simulink model "FullCarLateral"  (R2023b)
settings: Solver=FixedStepAuto  StartTime=0.0  StopTime=30  FixedStep=dt  MaxStep=0.001  RelTol=1e-3
model workspace (MAT data in the model file):
  AMU : Simulink.Signal (value not decoded)
  EPSILON : Simulink.Signal (value not decoded)
  FZO : Simulink.Signal (value not decoded)
  LCX : Simulink.Signal (value not decoded)
  LCY : Simulink.Signal (value not decoded)
  LCZ : Simulink.Signal (value not decoded)
  LEX : Simulink.Signal (value not decoded)
  LEY : Simulink.Signal (value not decoded)
  LFZO : Simulink.Signal (value not decoded)
  LHX : Simulink.Signal (value not decoded)
  LHY : Simulink.Signal (value not decoded)
  LKXKAPPA : Simulink.Signal (value not decoded)
  LKYALPHA : Simulink.Signal (value not decoded)
  LKYGAMMA : Simulink.Signal (value not decoded)
  LKZGAMMA : Simulink.Signal (value not decoded)
  LMR : Simulink.Signal (value not decoded)
  LMUV : Simulink.Signal (value not decoded)
  LMUX : Simulink.Signal (value not decoded)
  LMUXAST : Simulink.Signal (value not decoded)
  LMUXPRIME : Simulink.Signal (value not decoded)
  LMUY : Simulink.Signal (value not decoded)
  LMUYAST : Simulink.Signal (value not decoded)
  LMUYPRIME : Simulink.Signal (value not decoded)
  LMX : Simulink.Signal (value not decoded)
  LMY : Simulink.Signal (value not decoded)
  LS : Simulink.Signal (value not decoded)
  LT : Simulink.Signal (value not decoded)
  LVX : Simulink.Signal (value not decoded)
  LVY : Simulink.Signal (value not decoded)
  LVYKAPPA : Simulink.Signal (value not decoded)
  LXALPHA : Simulink.Signal (value not decoded)
  LYKAPPA : Simulink.Signal (value not decoded)
  PCX1 : Simulink.Signal (value not decoded)
  PCY1 : Simulink.Signal (value not decoded)
  PDX1 : Simulink.Signal (value not decoded)
  PDX2 : Simulink.Signal (value not decoded)
  PDX3 : Simulink.Signal (value not decoded)
  PDY1 : Simulink.Signal (value not decoded)
  PDY2 : Simulink.Signal (value not decoded)
  PDY3 : Simulink.Signal (value not decoded)
  PEX1 : Simulink.Signal (value not decoded)
  PEX2 : Simulink.Signal (value not decoded)
  PEX3 : Simulink.Signal (value not decoded)
  PEX4 : Simulink.Signal (value not decoded)
  PEY1 : Simulink.Signal (value not decoded)
  PEY2 : Simulink.Signal (value not decoded)
  PEY3 : Simulink.Signal (value not decoded)
  PEY4 : Simulink.Signal (value not decoded)
  PEY5 : Simulink.Signal (value not decoded)
  PHX1 : Simulink.Signal (value not decoded)
  PHX2 : Simulink.Signal (value not decoded)
  PHY1 : Simulink.Signal (value not decoded)
  PHY2 : Simulink.Signal (value not decoded)
  PKX1 : Simulink.Signal (value not decoded)
  PKX2 : Simulink.Signal (value not decoded)
  PKX3 : Simulink.Signal (value not decoded)
  PKY1 : Simulink.Signal (value not decoded)
  PKY2 : Simulink.Signal (value not decoded)
  PKY3 : Simulink.Signal (value not decoded)
  PKY4 : Simulink.Signal (value not decoded)
  PKY5 : Simulink.Signal (value not decoded)
  PKY6 : Simulink.Signal (value not decoded)
  PKY7 : Simulink.Signal (value not decoded)
  PVX1 : Simulink.Signal (value not decoded)
  PVX2 : Simulink.Signal (value not decoded)
  PVY1 : Simulink.Signal (value not decoded)
  PVY2 : Simulink.Signal (value not decoded)
  PVY3 : Simulink.Signal (value not decoded)
  PVY4 : Simulink.Signal (value not decoded)
  QBZ1 : Simulink.Signal (value not decoded)
  QBZ10 : Simulink.Signal (value not decoded)
  QBZ2 : Simulink.Signal (value not decoded)
  QBZ3 : Simulink.Signal (value not decoded)
  QBZ5 : Simulink.Signal (value not decoded)
  QBZ6 : Simulink.Signal (value not decoded)
  QBZ9 : Simulink.Signal (value not decoded)
  QCZ1 : Simulink.Signal (value not decoded)
  QDZ1 : Simulink.Signal (value not decoded)
  QDZ10 : Simulink.Signal (value not decoded)
  QDZ11 : Simulink.Signal (value not decoded)
  QDZ2 : Simulink.Signal (value not decoded)
  QDZ3 : Simulink.Signal (value not decoded)
  QDZ4 : Simulink.Signal (value not decoded)
  QDZ6 : Simulink.Signal (value not decoded)
  QDZ7 : Simulink.Signal (value not decoded)
  QDZ8 : Simulink.Signal (value not decoded)
  QDZ9 : Simulink.Signal (value not decoded)
  QEZ1 : Simulink.Signal (value not decoded)
  QEZ2 : Simulink.Signal (value not decoded)
  QEZ3 : Simulink.Signal (value not decoded)
  QEZ4 : Simulink.Signal (value not decoded)
  QEZ5 : Simulink.Signal (value not decoded)
  QHZ1 : Simulink.Signal (value not decoded)
  QHZ2 : Simulink.Signal (value not decoded)
  QHZ3 : Simulink.Signal (value not decoded)
  QHZ4 : Simulink.Signal (value not decoded)
  QSX1 : Simulink.Signal (value not decoded)
  QSX2 : Simulink.Signal (value not decoded)
  QSX3 : Simulink.Signal (value not decoded)
  QX1 : Simulink.Signal (value not decoded)
  QX2 : Simulink.Signal (value not decoded)
  QX3 : Simulink.Signal (value not decoded)
  QX4 : Simulink.Signal (value not decoded)
  QX5 : Simulink.Signal (value not decoded)
  QX6 : Simulink.Signal (value not decoded)
  RBX1 : Simulink.Signal (value not decoded)
  RBX2 : Simulink.Signal (value not decoded)
  RBX3 : Simulink.Signal (value not decoded)
  RBY1 : Simulink.Signal (value not decoded)
  RBY2 : Simulink.Signal (value not decoded)
  RBY3 : Simulink.Signal (value not decoded)
  RBY4 : Simulink.Signal (value not decoded)
  RCX1 : Simulink.Signal (value not decoded)
  RCY1 : Simulink.Signal (value not decoded)
  REX1 : Simulink.Signal (value not decoded)
  REX2 : Simulink.Signal (value not decoded)
  REY1 : Simulink.Signal (value not decoded)
  REY2 : Simulink.Signal (value not decoded)
  RHX1 : Simulink.Signal (value not decoded)
  RHY1 : Simulink.Signal (value not decoded)
  RHY2 : Simulink.Signal (value not decoded)
  RO : Simulink.Signal (value not decoded)
  RVY1 : Simulink.Signal (value not decoded)
  RVY2 : Simulink.Signal (value not decoded)
  RVY3 : Simulink.Signal (value not decoded)
  RVY4 : Simulink.Signal (value not decoded)
  RVY5 : Simulink.Signal (value not decoded)
  RVY6 : Simulink.Signal (value not decoded)
  SSZ1 : Simulink.Signal (value not decoded)
  SSZ2 : Simulink.Signal (value not decoded)
  SSZ3 : Simulink.Signal (value not decoded)
  SSZ4 : Simulink.Signal (value not decoded)
  VCX : Simulink.Signal (value not decoded)
  ZETA0 : Simulink.Signal (value not decoded)
  ZETA1 : Simulink.Signal (value not decoded)
  ZETA2 : Simulink.Signal (value not decoded)
  ZETA3 : Simulink.Signal (value not decoded)
  ZETA4 : Simulink.Signal (value not decoded)
  ZETA5 : Simulink.Signal (value not decoded)
  ZETA6 : Simulink.Signal (value not decoded)
  ZETA7 : Simulink.Signal (value not decoded)
  ZETA8 : Simulink.Signal (value not decoded)
values from neighbouring files (symbols this model uses):
  A = load('PSS LATERAL FORCE COEFFS.mat').A    [FullCarLateralParams.m]
  B = load('PSS ALIGNING TORQUE COEFFS.mat').B    [FullCarLateralParams.m]
  b = 0.085    [FullCarLateralParams.m]
  C = load('COMBINED OVERTURNING MOMENT COEFFS.mat').C    [FullCarLateralParams.m]
  c_roll = 0.1    [FullCarLateralParams.m]
  cD = 1.23    [FullCarLateralParams.m]
  cL = 3.71    [FullCarLateralParams.m]
  D = load('PLS LONGITUDINAL FORCE COEFFS.mat').D    [FullCarLateralParams.m]
  dt = 0.001    [FullCarLateralParams.m]
  E = load('COMBINED LONGITUDINAL FORCE COEFFS.mat').E    [FullCarLateralParams.m]
  e_FL = atan(tf/lf)    [FullCarLateralParams.m]
  e_FR = atan(lf/tf)    [FullCarLateralParams.m]
  e_RL = atan(lr/tr)    [FullCarLateralParams.m]
  e_RR = atan(tr/lr)    [FullCarLateralParams.m]
  F = load('COMBINED LATERAL FORCE COEFFS.mat').F    [FullCarLateralParams.m]
  frontalA = 1    [FullCarLateralParams.m]
  g = 9.81    [FullCarLateralParams.m]
  G = load('COMBINED ALIGNING TORQUE COEFFS.mat').G    [FullCarLateralParams.m]
  gearboxEff = 0.95    [FullCarLateralParams.m]
  GR = 11.86    [FullCarLateralParams.m]
  hCG = 0.2    [FullCarLateralParams.m]
  Ix_wheel = (0.07829 + Ix_motor*GR*GR) * Ix_wheel_factor    (= 0.1168307304)    [FullCarLateralParams.m]
  Iz_vehicle = 125    [FullCarLateralParams.m]
  lf = wb - lr    (= 0.755)    [FullCarLateralParams.m]
  lowpassT = 0.05    [FullCarLateralParams.m]
  lr = 0.78    [FullCarLateralParams.m]
  m = 250    [FullCarLateralParams.m]
  motorOmegaLimit = 2094    [FullCarLateralParams.m]
  R_FL = sqrt(tf^2 + lf^2)    [FullCarLateralParams.m]
  R_FR = R_FL    [FullCarLateralParams.m]
  R_RL = sqrt(tr^2 + lr^2)    [FullCarLateralParams.m]
  R_RR = R_RL    [FullCarLateralParams.m]
  R_wheel = 0.2    [FullCarLateralParams.m]
  rho = 1.293    [FullCarLateralParams.m]
  tireFactor_X_Accel = 0.6    [FullCarLateralParams.m]
  tireFactor_X_Brake = 0.6    [FullCarLateralParams.m]
  tireFactor_Y = 1    [FullCarLateralParams.m]
  TLLTD = 0.5    [FullCarLateralParams.m]
  tr = trackWidth / 2    (= 0.6)    [FullCarLateralParams.m]
  trackWidth = 1.2    [FullCarLateralParams.m]
  wb = 1.535    [FullCarLateralParams.m]
  wheelSideBrakeFactor = 1    [FullCarLateralParams.m]
undefined symbols (not defined in the file or in its folder): trackReference
libraries: simulink_extras x11, eeGeneralControl x3, slpidlib x2, simulink x2
(part 3 of 6)

== system FullCarLateral/Car/Tire Model Pacejka 5.2/Subsystem1 ==
  FX : Inport
  If : If  IfExpression=u1 >= 0
  If Action Subsystem : Subsystem  TreatAsAtomicUnit=on
  If Action Subsystem1 : Subsystem  TreatAsAtomicUnit=on
  Merge : Merge
  FX_W FR : Outport
  wires:
  If Action Subsystem1/1(Out1) -> Merge/2
  If Action Subsystem/1(Out1) -> Merge/1
  If/2 -> If Action Subsystem1/Action
  Merge/1 -> FX_W FR/1  "FX_W FL"
  FX/1 -> If Action Subsystem/1(FX), If Action Subsystem1/1(FX), If/1
  If/1 -> If Action Subsystem/Action

== system FullCarLateral/Car/Tire Model Pacejka 5.2/Subsystem2 ==
  FX : Inport
  If : If  IfExpression=u1 >= 0
  If Action Subsystem : Subsystem  TreatAsAtomicUnit=on
  If Action Subsystem1 : Subsystem  TreatAsAtomicUnit=on
  Merge : Merge
  FX_W RL : Outport
  wires:
  If/1 -> If Action Subsystem/Action
  FX/1 -> If/1, If Action Subsystem1/1(FX), If Action Subsystem/1(FX)
  Merge/1 -> FX_W RL/1  "FX_W FL"
  If/2 -> If Action Subsystem1/Action
  If Action Subsystem/1(Out1) -> Merge/1
  If Action Subsystem1/1(Out1) -> Merge/2

== system FullCarLateral/Car/Tire Model Pacejka 5.2/Subsystem3 ==
  FX : Inport
  If : If  IfExpression=u1 >= 0
  If Action Subsystem : Subsystem  TreatAsAtomicUnit=on
  If Action Subsystem1 : Subsystem  TreatAsAtomicUnit=on
  Merge : Merge
  FX_W RR : Outport
  wires:
  If Action Subsystem1/1(Out1) -> Merge/2
  If Action Subsystem/1(Out1) -> Merge/1
  If/2 -> If Action Subsystem1/Action
  Merge/1 -> FX_W RR/1  "FX_W FL"
  FX/1 -> If Action Subsystem/1(FX), If Action Subsystem1/1(FX), If/1
  If/1 -> If Action Subsystem/Action

== system FullCarLateral/Car/Wheel Dynamics/Subsystem ==
  FX : Inport
  FY : Inport  Port=2
  Add : Sum
  Product : Product
  Product1 : Product
  Product2 : Product
  Sign : Signum
  Sqrt : Sqrt
  F NET : Outport
  wires:
  FX/1 -> Sign/1, Product/2, Product/1
  FY/1 -> Product1/1, Product1/2
  Product/1 -> Add/1
  Product1/1 -> Add/2
  Add/1 -> Sqrt/1
  Sqrt/1 -> Product2/2
  Sign/1 -> Product2/1
  Product2/1 -> F NET/1

== system FullCarLateral/Car/Wheel Dynamics/Subsystem1 ==
  FX : Inport
  FY : Inport  Port=2
  Add : Sum
  Product : Product
  Product1 : Product
  Product2 : Product
  Sign : Signum
  Sqrt : Sqrt
  F NET : Outport
  wires:
  Product2/1 -> F NET/1
  Sign/1 -> Product2/1
  Sqrt/1 -> Product2/2
  Add/1 -> Sqrt/1
  Product1/1 -> Add/2
  Product/1 -> Add/1
  FY/1 -> Product1/2, Product1/1
  FX/1 -> Product/1, Product/2, Sign/1

== system FullCarLateral/Car/Wheel Dynamics/Subsystem2 ==
  FX : Inport
  FY : Inport  Port=2
  Add : Sum
  Product : Product
  Product1 : Product
  Product2 : Product
  Sign : Signum
  Sqrt : Sqrt
  F NET : Outport
  wires:
  FX/1 -> Sign/1, Product/2, Product/1
  FY/1 -> Product1/1, Product1/2
  Product/1 -> Add/1
  Product1/1 -> Add/2
  Add/1 -> Sqrt/1
  Sqrt/1 -> Product2/2
  Sign/1 -> Product2/1
  Product2/1 -> F NET/1

== system FullCarLateral/Car/Wheel Dynamics/Subsystem3 ==
  FX : Inport
  FY : Inport  Port=2
  Add : Sum
  Product : Product
  Product1 : Product
  Product2 : Product
  Sign : Signum
  Sqrt : Sqrt
  F NET : Outport
  wires:
  Product2/1 -> F NET/1
  Sign/1 -> Product2/1
  Sqrt/1 -> Product2/2
  Add/1 -> Sqrt/1
  Product1/1 -> Add/2
  Product/1 -> Add/1
  FY/1 -> Product1/2, Product1/1
  FX/1 -> Product/1, Product/2, Sign/1

== system FullCarLateral/Car/Wheel Dynamics/Subsystem4 ==
  Requested Motor Torque : Inport
  FX Resistance : Inport  Port=2
  Long Corner Vel : Inport  Port=3
  Accel. or Rolling No Slip : Subsystem  TreatAsAtomicUnit=on
  Braking : Subsystem  TreatAsAtomicUnit=on
  Constant : Constant  Value=0
  If : If  IfExpression=u1 >= 0
  Merge : Merge
  Merge1 : Merge
  Switch : Switch  Criteria=u2 > Threshold  SaturateOnIntegerOverflow=off  InputSameDT=off
  Wheel Omega : Outport
  Constrained Motor Torque : Outport  Port=2
  wires:
  Requested Motor Torque/1 -> Braking/1(Requested Motor Torque), Accel. or Rolling No Slip/1(Requested Motor Torque), If/1
  If/1 -> Accel. or Rolling No Slip/Action
  If/2 -> Braking/Action
  FX Resistance/1 -> Braking/2(FX Resistance), Accel. or Rolling No Slip/2(FX Resistance)
  Long Corner Vel/1 -> Accel. or Rolling No Slip/3(Long Corner Vel)
  Accel. or Rolling No Slip/1(Wheel Omega) -> Merge/1
  Braking/1(Wheel Omega) -> Merge/2
  Accel. or Rolling No Slip/2(Constrained Motor Torque) -> Merge1/1
  Braking/2(Constrained Motor Torque) -> Merge1/2
  Merge1/1 -> Constrained Motor Torque/1
  Merge/1 -> Switch/2, Switch/1
  Switch/1 -> Wheel Omega/1
  Constant/1 -> Switch/3

== system FullCarLateral/Car/Wheel Dynamics/Subsystem5 ==
  Requested Motor Torque : Inport
  FX Resistance : Inport  Port=2
  Long Corner Vel : Inport  Port=3
  Accel. or Rolling No Slip : Subsystem  TreatAsAtomicUnit=on
  Braking : Subsystem  TreatAsAtomicUnit=on
  Constant : Constant  Value=0
  If : If  IfExpression=u1 >= 0
  Merge : Merge
  Merge1 : Merge
  Switch : Switch  Criteria=u2 > Threshold  SaturateOnIntegerOverflow=off  InputSameDT=off
  Wheel Omega : Outport
  Constrained Motor Torque : Outport  Port=2
  wires:
  Merge1/1 -> Constrained Motor Torque/1
  Braking/2(Constrained Motor Torque) -> Merge1/2
  Accel. or Rolling No Slip/2(Constrained Motor Torque) -> Merge1/1
  Braking/1(Wheel Omega) -> Merge/2
  Accel. or Rolling No Slip/1(Wheel Omega) -> Merge/1
  Long Corner Vel/1 -> Accel. or Rolling No Slip/3(Long Corner Vel)
  FX Resistance/1 -> Accel. or Rolling No Slip/2(FX Resistance), Braking/2(FX Resistance)
  If/2 -> Braking/Action
  If/1 -> Accel. or Rolling No Slip/Action
  Requested Motor Torque/1 -> If/1, Accel. or Rolling No Slip/1(Requested Motor Torque), Braking/1(Requested Motor Torque)
  Constant/1 -> Switch/3
  Merge/1 -> Switch/2, Switch/1
  Switch/1 -> Wheel Omega/1

== system FullCarLateral/Car/Wheel Dynamics/Subsystem6 ==
  Requested Motor Torque : Inport
  FX Resistance : Inport  Port=2
  Long Corner Vel : Inport  Port=3
  Accel. or Rolling No Slip : Subsystem  TreatAsAtomicUnit=on
  Braking : Subsystem  TreatAsAtomicUnit=on
  Constant : Constant  Value=0
  If : If  IfExpression=u1 >= 0
  Merge : Merge
  Merge1 : Merge
  Switch : Switch  Criteria=u2 > Threshold  SaturateOnIntegerOverflow=off  InputSameDT=off
  Wheel Omega : Outport
  Constrained Motor Torque : Outport  Port=2
  wires:
  Requested Motor Torque/1 -> Braking/1(Requested Motor Torque), Accel. or Rolling No Slip/1(Requested Motor Torque), If/1
  If/1 -> Accel. or Rolling No Slip/Action
  If/2 -> Braking/Action
  FX Resistance/1 -> Braking/2(FX Resistance), Accel. or Rolling No Slip/2(FX Resistance)
  Long Corner Vel/1 -> Accel. or Rolling No Slip/3(Long Corner Vel)
  Accel. or Rolling No Slip/1(Wheel Omega) -> Merge/1
  Braking/1(Wheel Omega) -> Merge/2
  Accel. or Rolling No Slip/2(Constrained Motor Torque) -> Merge1/1
  Braking/2(Constrained Motor Torque) -> Merge1/2
  Merge1/1 -> Constrained Motor Torque/1
  Constant/1 -> Switch/3
  Merge/1 -> Switch/2, Switch/1
  Switch/1 -> Wheel Omega/1

== system FullCarLateral/Car/Wheel Dynamics/Subsystem7 ==
  Requested Motor Torque : Inport
  FX Resistance : Inport  Port=2
  Long Corner Vel : Inport  Port=3
  Accel. or Rolling No Slip : Subsystem  TreatAsAtomicUnit=on
  Braking : Subsystem  TreatAsAtomicUnit=on
  Constant : Constant  Value=0
  If : If  IfExpression=u1 >= 0
  Merge : Merge
  Merge1 : Merge
  Switch : Switch  Criteria=u2 > Threshold  SaturateOnIntegerOverflow=off  InputSameDT=off
  Wheel Omega : Outport
  Constrained Motor Torque : Outport  Port=2
  wires:
  Merge1/1 -> Constrained Motor Torque/1
  Braking/2(Constrained Motor Torque) -> Merge1/2
  Accel. or Rolling No Slip/2(Constrained Motor Torque) -> Merge1/1
  Braking/1(Wheel Omega) -> Merge/2
  Accel. or Rolling No Slip/1(Wheel Omega) -> Merge/1
  Long Corner Vel/1 -> Accel. or Rolling No Slip/3(Long Corner Vel)
  FX Resistance/1 -> Accel. or Rolling No Slip/2(FX Resistance), Braking/2(FX Resistance)
  If/2 -> Braking/Action
  If/1 -> Accel. or Rolling No Slip/Action
  Requested Motor Torque/1 -> If/1, Accel. or Rolling No Slip/1(Requested Motor Torque), Braking/1(Requested Motor Torque)
  Constant/1 -> Switch/3
  Merge/1 -> Switch/2, Switch/1
  Switch/1 -> Wheel Omega/1

== system FullCarLateral/Car/Wheel Dynamics/Wheel Omega Calc FL1 ==
  Requested Motor Torque : Inport
  FX Resistance : Inport  Port=2
  Add3 : Sum
  Apply Motor Omega Limit Constraint : Subsystem  TreatAsAtomicUnit=on
  Constant12 : Constant  Value=b
  Constant16 : Constant  Value=GR
  Constant20 : Constant  Value=R_wheel
  Data Store Read2 : DataStoreRead  DataStoreName=wheelOmegaFL  IndexOptions=Index vector (dialog)  Indices=1  OutputSizes=1
  Divide : Product  Inputs=*/
  Fcn3 : Fcn  Expr=u/Ix_wheel
  Gain : Gain  Gain=wheelSideBrakeFactor
  Gain14 : Gain  Gain=gearboxEff
  Gain15 : Gain  Gain=dt
  Gain16 : Gain  Gain=GR
  If3 : If  IfExpression=u1 > motorOmegaLimit
  Memory2 : Memory
  No Omega Limit Constraint : Subsystem  TreatAsAtomicUnit=on
  Product15 : Product
  Product16 : Product
  Product20 : Product
  Subtract5 : Sum  Inputs=+--
  Switch : Switch  Criteria=u2 > Threshold  SaturateOnIntegerOverflow=off  InputSameDT=off
  Terminator : Terminator
  wires:
  Product16/1 -> Gain14/1
  Product20/1 -> Subtract5/2
  Requested Motor Torque/1 -> No Omega Limit Constraint/2(Unconstrained Requested Motor Torque), Apply Motor Omega Limit Constraint/1(Requested Motor Torque), Product16/1
  Add3/1 -> Gain16/1, No Omega Limit Constraint/1(Wheel Omega), Product15/2  "Wheel Omega"
  Data Store Read2/1 -> Add3/2  "Previous Wheel Omega"
  Memory2/1 -> Gain15/1
  Subtract5/1 -> Fcn3/1
  Constant20/1 -> Divide/2, Product20/2
  Gain15/1 -> Add3/1  "Delta Wheel Omega"
  Fcn3/1 -> Memory2/1  "Wheel Omega Dot"
  If3/2 -> No Omega Limit Constraint/Action
  Product15/1 -> Subtract5/3
  Constant12/1 -> Product15/1
  Gain14/1 -> Divide/1, Subtract5/1  "Requested Wheel Output Torque"
  Constant16/1 -> Product16/2
  If3/1 -> Apply Motor Omega Limit Constraint/Action
  Gain16/1 -> If3/1  "Motor Omega"
  Switch/1 -> Product20/1, Apply Motor Omega Limit Constraint/2(F_Roll)
  FX Resistance/1 -> Switch/1, Switch/2, Gain/1
  Gain/1 -> Switch/3
  Divide/1 -> Terminator/1  "Linear Force From Motor Torque FL"

== system FullCarLateral/Car/Wheel Dynamics/Wheel Omega Calc FR1 ==
  Requested Motor Torque : Inport
  FX Resistance : Inport  Port=2
  Add3 : Sum
  Apply Motor Omega Limit Constraint : Subsystem  TreatAsAtomicUnit=on
  Constant12 : Constant  Value=b
  Constant16 : Constant  Value=GR
  Constant20 : Constant  Value=R_wheel
  Data Store Read2 : DataStoreRead  DataStoreName=wheelOmegaFR  IndexOptions=Index vector (dialog)  Indices=1  OutputSizes=1
  Fcn3 : Fcn  Expr=u/Ix_wheel
  Gain1 : Gain  Gain=wheelSideBrakeFactor
  Gain14 : Gain  Gain=gearboxEff
  Gain15 : Gain  Gain=dt
  Gain16 : Gain  Gain=GR
  If3 : If  IfExpression=u1 > motorOmegaLimit
  Memory2 : Memory
  No Omega Limit Constraint : Subsystem  TreatAsAtomicUnit=on
  Product15 : Product
  Product16 : Product
  Product20 : Product
  Subtract5 : Sum  Inputs=+--
  Switch1 : Switch  Criteria=u2 > Threshold  SaturateOnIntegerOverflow=off  InputSameDT=off
  wires:
  Gain16/1 -> If3/1  "Motor Omega"
  If3/1 -> Apply Motor Omega Limit Constraint/Action
  Constant16/1 -> Product16/2
  Gain14/1 -> Subtract5/1  "Requested Wheel Output Torque"
  Constant12/1 -> Product15/1
  Product15/1 -> Subtract5/3
  If3/2 -> No Omega Limit Constraint/Action
  Fcn3/1 -> Memory2/1  "Wheel Omega Dot"
  Gain15/1 -> Add3/1  "Delta Wheel Omega"
  Constant20/1 -> Product20/2
  Subtract5/1 -> Fcn3/1
  Memory2/1 -> Gain15/1
  Data Store Read2/1 -> Add3/2  "Previous Wheel Omega"
  Add3/1 -> Product15/2, No Omega Limit Constraint/1(Wheel Omega), Gain16/1  "Wheel Omega"
  Requested Motor Torque/1 -> Product16/1, Apply Motor Omega Limit Constraint/1(Requested Motor Torque), No Omega Limit Constraint/2(Unconstrained Requested Motor Torque)
  Product20/1 -> Subtract5/2
  Product16/1 -> Gain14/1
  Gain1/1 -> Switch1/3
  FX Resistance/1 -> Gain1/1, Switch1/2, Switch1/1
  Switch1/1 -> Product20/1, Apply Motor Omega Limit Constraint/2(F_Roll)

== system FullCarLateral/Car/Wheel Dynamics/Wheel Omega Calc RL1 ==
  Requested Motor Torque : Inport
  FX Resistance : Inport  Port=2
  Add3 : Sum
  Apply Motor Omega Limit Constraint : Subsystem  TreatAsAtomicUnit=on
  Constant12 : Constant  Value=b
  Constant16 : Constant  Value=GR
  Constant20 : Constant  Value=R_wheel
  Data Store Read2 : DataStoreRead  DataStoreName=wheelOmegaRL  IndexOptions=Index vector (dialog)  Indices=1  OutputSizes=1
  Fcn3 : Fcn  Expr=u/Ix_wheel
  Gain : Gain  Gain=wheelSideBrakeFactor
  Gain14 : Gain  Gain=gearboxEff
  Gain15 : Gain  Gain=dt
  Gain16 : Gain  Gain=GR
  If3 : If  IfExpression=u1 > motorOmegaLimit
  Memory2 : Memory
  No Omega Limit Constraint : Subsystem  TreatAsAtomicUnit=on
  Product15 : Product
  Product16 : Product
  Product20 : Product
  Subtract5 : Sum  Inputs=+--
  Switch : Switch  Criteria=u2 > Threshold  SaturateOnIntegerOverflow=off  InputSameDT=off
  wires:
  Product16/1 -> Gain14/1
  Product20/1 -> Subtract5/2
  Requested Motor Torque/1 -> No Omega Limit Constraint/2(Unconstrained Requested Motor Torque), Apply Motor Omega Limit Constraint/1(Requested Motor Torque), Product16/1
  Add3/1 -> Gain16/1, No Omega Limit Constraint/1(Wheel Omega), Product15/2  "Wheel Omega"
  Data Store Read2/1 -> Add3/2  "Previous Wheel Omega"
  Memory2/1 -> Gain15/1
  Subtract5/1 -> Fcn3/1
  Constant20/1 -> Product20/2
  Gain15/1 -> Add3/1  "Delta Wheel Omega"
  Fcn3/1 -> Memory2/1  "Wheel Omega Dot"
  If3/2 -> No Omega Limit Constraint/Action
  Product15/1 -> Subtract5/3
  Constant12/1 -> Product15/1
  Gain14/1 -> Subtract5/1  "Requested Wheel Output Torque"
  Constant16/1 -> Product16/2
  If3/1 -> Apply Motor Omega Limit Constraint/Action
  Gain16/1 -> If3/1  "Motor Omega"
  Gain/1 -> Switch/3
  FX Resistance/1 -> Switch/1, Gain/1, Switch/2
  Switch/1 -> Apply Motor Omega Limit Constraint/2(F_Roll), Product20/1

== system FullCarLateral/Car/Wheel Dynamics/Wheel Omega Calc RR1 ==
  Requested Motor Torque : Inport
  FX Resistance : Inport  Port=2
  Add3 : Sum
  Apply Motor Omega Limit Constraint : Subsystem  TreatAsAtomicUnit=on
  Constant12 : Constant  Value=b
  Constant16 : Constant  Value=GR
  Constant20 : Constant  Value=R_wheel
  Data Store Read2 : DataStoreRead  DataStoreName=wheelOmegaRR  IndexOptions=Index vector (dialog)  Indices=1  OutputSizes=1
  Fcn3 : Fcn  Expr=u/Ix_wheel
  Gain : Gain  Gain=wheelSideBrakeFactor
  Gain14 : Gain  Gain=gearboxEff
  Gain15 : Gain  Gain=dt
  Gain16 : Gain  Gain=GR
  If3 : If  IfExpression=u1 > motorOmegaLimit
  Memory2 : Memory
  No Omega Limit Constraint : Subsystem  TreatAsAtomicUnit=on
  Product15 : Product
  Product16 : Product
  Product20 : Product
  Subtract5 : Sum  Inputs=+--
  Switch : Switch  Criteria=u2 > Threshold  SaturateOnIntegerOverflow=off  InputSameDT=off
  wires:
  Gain16/1 -> If3/1  "Motor Omega"
  If3/1 -> Apply Motor Omega Limit Constraint/Action
  Constant16/1 -> Product16/2
  Gain14/1 -> Subtract5/1  "Requested Wheel Output Torque"
  Constant12/1 -> Product15/1
  Product15/1 -> Subtract5/3
  If3/2 -> No Omega Limit Constraint/Action
  Fcn3/1 -> Memory2/1  "Wheel Omega Dot"
  Gain15/1 -> Add3/1  "Delta Wheel Omega"
  Constant20/1 -> Product20/2
  Subtract5/1 -> Fcn3/1
  Memory2/1 -> Gain15/1
  Data Store Read2/1 -> Add3/2  "Previous Wheel Omega"
  Add3/1 -> Product15/2, No Omega Limit Constraint/1(Wheel Omega), Gain16/1  "Wheel Omega"
  Requested Motor Torque/1 -> Product16/1, Apply Motor Omega Limit Constraint/1(Requested Motor Torque), No Omega Limit Constraint/2(Unconstrained Requested Motor Torque)
  Product20/1 -> Subtract5/2
  Product16/1 -> Gain14/1
  Gain/1 -> Switch/3
  FX Resistance/1 -> Switch/1, Gain/1, Switch/2
  Switch/1 -> Product20/1, Apply Motor Omega Limit Constraint/2(F_Roll)

== system FullCarLateral/Car/Longitudinal Slip/Longitudinal Slip Calc FL/Accel. Calc ==
  Corner Speed : Inport
  Wheel Omega1 : Inport  Port=2
  Action Port : ActionPort  ActionPortLabel=if(u1 > 0)
  Add : Sum  Commented=on
  Constant : Constant  Value=R_wheel
  Constant1 : Constant  Value=inf
  Constant2 : Constant
  Constant3 : Constant  Value=0
  Constant4 : Constant  Commented=on
  Divide : Product  Inputs=*/
  From : From  Commented=on  GotoTag=SL
  From1 : From  Commented=on  GotoTag=SS
  Product : Product
  Product3 : Product  Commented=on
  Product4 : Product  Commented=on
  Sqrt : Sqrt  Commented=on
  Subtract : Sum  Inputs=+-
  Switch : Switch  Criteria=u2 ~= 0  SaturateOnIntegerOverflow=off  InputSameDT=off
  Switch1 : Switch  Criteria=u2 > Threshold  Threshold=1  SaturateOnIntegerOverflow=off  InputSameDT=off
  Switch2 : Switch  Commented=on  Criteria=u2 > Threshold  Threshold=1  SaturateOnIntegerOverflow=off  InputSameDT=off
  Switch3 : Switch  Criteria=u2 > Threshold  SaturateOnIntegerOverflow=off  InputSameDT=off
  SL : Outport
  wires:
  Switch/1 -> Divide/2
  Constant1/1 -> Switch/3
  Subtract/1 -> Divide/1
  Corner Speed/1 -> Subtract/2
  Add/1 -> Sqrt/1
  Sqrt/1 -> Switch2/2, Switch2/1
  Constant4/1 -> Switch2/3
  From/1 -> Product3/1, Product3/2
  Product4/1 -> Add/2
  From1/1 -> Product4/2, Product4/1
  Product3/1 -> Add/1
  Constant/1 -> Product/2
  Wheel Omega1/1 -> Product/1
  Product/1 -> Subtract/1, Switch/1, Switch/2  "Omega * Rw"
  Constant2/1 -> Switch1/1
  Divide/1 -> Switch3/2, Switch3/1  "Longitudinal Slip (SL)"
  Constant3/1 -> Switch3/3
  Switch3/1 -> Switch1/3, Switch1/2
  Switch1/1 -> SL/1

== system FullCarLateral/Car/Longitudinal Slip/Longitudinal Slip Calc FL/Brake Calc ==
  Wheel Omega : Inport
  Corner Speed : Inport  Port=2
  Action Port : ActionPort  ActionPortLabel=elseif(u1 < 0)
  Abs : Abs  SaturateOnIntegerOverflow=off
  Abs1 : Abs  SaturateOnIntegerOverflow=off
  Add : Sum  Commented=on
  Constant : Constant  Value=R_wheel
  Constant1 : Constant  Value=-1
  Constant2 : Constant  Commented=on  Value=-1
  Constant3 : Constant  Commented=on
  Divide : Product  Inputs=*/
  From : From  Commented=on  GotoTag=SL
  From1 : From  Commented=on  GotoTag=SS
  Gain : Gain  Gain=-1
  Goto : Goto  Commented=on  GotoTag=SL
  Goto1 : Goto  Commented=on  GotoTag=SS
  Product : Product
  Product3 : Product  Commented=on
  Product4 : Product  Commented=on
  Product5 : Product  Commented=on
  Sqrt : Sqrt  Commented=on
  Subtract : Sum  Inputs=+-
  Switch : Switch  Criteria=u2 > Threshold  Threshold=1  SaturateOnIntegerOverflow=off  InputSameDT=off
  Switch1 : Switch  Commented=on  Criteria=u2 > Threshold  Threshold=1  SaturateOnIntegerOverflow=off  InputSameDT=off
  SL : Outport
  wires:
  Divide/1 -> Switch/3, Abs/1  "Longitudinal Slip (SL)"
  Subtract/1 -> Divide/1
  Product/1 -> Subtract/1  "Omega * Rw"
  Corner Speed/1 -> Subtract/2, Divide/2
  Wheel Omega/1 -> Product/1
  Constant/1 -> Product/2
  Abs/1 -> Switch/2
  Switch/1 -> Abs1/1, Goto/1
  From/1 -> Product3/1, Product3/2
  From1/1 -> Product4/2, Product4/1
  Product3/1 -> Add/1
  Product4/1 -> Add/2
  Add/1 -> Sqrt/1
  Constant2/1 -> Product5/2
  Sqrt/1 -> Switch1/2, Switch1/1
  Constant3/1 -> Switch1/3
  Switch1/1 -> Product5/1
  Constant1/1 -> Switch/1
  Gain/1 -> SL/1
  Abs1/1 -> Gain/1

== system FullCarLateral/Car/Longitudinal Slip/Longitudinal Slip Calc FL/If Action Subsystem ==
  in : Inport
  Action Port : ActionPort  ActionPortLabel=else
  Out1 : Outport
  wires:
  in/1 -> Out1/1

== system FullCarLateral/Car/Longitudinal Slip/Longitudinal Slip Calc FL1/Accel. Calc ==
  Corner Speed : Inport
  Wheel Omega1 : Inport  Port=2
  Action Port : ActionPort  ActionPortLabel=if(u1 > 0)
  Add : Sum  Commented=on
  Constant : Constant  Value=R_wheel
  Constant1 : Constant  Value=inf
  Constant2 : Constant
  Constant3 : Constant  Value=0
  Constant4 : Constant  Commented=on
  Divide : Product  Inputs=*/
  From : From  Commented=on  GotoTag=SL
  From1 : From  Commented=on  GotoTag=SS
  Product : Product
  Product3 : Product  Commented=on
  Product4 : Product  Commented=on
  Sqrt : Sqrt  Commented=on
  Subtract : Sum  Inputs=+-
  Switch : Switch  Criteria=u2 ~= 0  SaturateOnIntegerOverflow=off  InputSameDT=off
  Switch1 : Switch  Criteria=u2 > Threshold  Threshold=1  SaturateOnIntegerOverflow=off  InputSameDT=off
  Switch2 : Switch  Commented=on  Criteria=u2 > Threshold  Threshold=1  SaturateOnIntegerOverflow=off  InputSameDT=off
  Switch3 : Switch  Criteria=u2 > Threshold  SaturateOnIntegerOverflow=off  InputSameDT=off
  SL : Outport
  wires:
  Switch1/1 -> SL/1
  Switch3/1 -> Switch1/2, Switch1/3
  Constant3/1 -> Switch3/3
  Divide/1 -> Switch3/1, Switch3/2  "Longitudinal Slip (SL)"
  Constant2/1 -> Switch1/1
  Product/1 -> Switch/2, Switch/1, Subtract/1  "Omega * Rw"
  Wheel Omega1/1 -> Product/1
  Constant/1 -> Product/2
  Product3/1 -> Add/1
  From1/1 -> Product4/1, Product4/2
  Product4/1 -> Add/2
  From/1 -> Product3/2, Product3/1
  Constant4/1 -> Switch2/3
  Sqrt/1 -> Switch2/1, Switch2/2
  Add/1 -> Sqrt/1
  Corner Speed/1 -> Subtract/2
  Subtract/1 -> Divide/1
  Constant1/1 -> Switch/3
  Switch/1 -> Divide/2

== system FullCarLateral/Car/Longitudinal Slip/Longitudinal Slip Calc FL1/Brake Calc ==
  Wheel Omega : Inport
  Corner Speed : Inport  Port=2
  Action Port : ActionPort  ActionPortLabel=elseif(u1 < 0)
  Abs : Abs  SaturateOnIntegerOverflow=off
  Abs1 : Abs  SaturateOnIntegerOverflow=off
  Add : Sum  Commented=on
  Constant : Constant  Value=R_wheel
  Constant1 : Constant  Value=-1
  Constant2 : Constant  Commented=on  Value=-1
  Constant3 : Constant  Commented=on
  Divide : Product  Inputs=*/
  From : From  Commented=on  GotoTag=SL
  From1 : From  Commented=on  GotoTag=SS
  Gain : Gain  Gain=-1
  Goto : Goto  Commented=on  GotoTag=SL
  Goto1 : Goto  Commented=on  GotoTag=SS
  Product : Product
  Product3 : Product  Commented=on
  Product4 : Product  Commented=on
  Product5 : Product  Commented=on
  Sqrt : Sqrt  Commented=on
  Subtract : Sum  Inputs=+-
  Switch : Switch  Criteria=u2 > Threshold  Threshold=1  SaturateOnIntegerOverflow=off  InputSameDT=off
  Switch1 : Switch  Commented=on  Criteria=u2 > Threshold  Threshold=1  SaturateOnIntegerOverflow=off  InputSameDT=off
  SL : Outport
  wires:
  Abs1/1 -> Gain/1
  Gain/1 -> SL/1
  Constant1/1 -> Switch/1
  Switch1/1 -> Product5/1
  Constant3/1 -> Switch1/3
  Sqrt/1 -> Switch1/1, Switch1/2
  Constant2/1 -> Product5/2
  Add/1 -> Sqrt/1
  Product4/1 -> Add/2
  Product3/1 -> Add/1
  From1/1 -> Product4/1, Product4/2
  From/1 -> Product3/2, Product3/1
  Switch/1 -> Goto/1, Abs1/1
  Abs/1 -> Switch/2
  Constant/1 -> Product/2
  Wheel Omega/1 -> Product/1
  Corner Speed/1 -> Divide/2, Subtract/2
  Product/1 -> Subtract/1  "Omega * Rw"
  Subtract/1 -> Divide/1
  Divide/1 -> Abs/1, Switch/3  "Longitudinal Slip (SL)"

== system FullCarLateral/Car/Longitudinal Slip/Longitudinal Slip Calc FL1/If Action Subsystem ==
  Corner Speed : Inport
  Action Port : ActionPort  ActionPortLabel=else
  Out1 : Outport
  wires:
  Corner Speed/1 -> Out1/1

== system FullCarLateral/Car/Longitudinal Slip/Longitudinal Slip Calc FL2/Accel. Calc ==
  Corner Speed : Inport
  Wheel Omega1 : Inport  Port=2
  Action Port : ActionPort  ActionPortLabel=if(u1 > 0)
  Add : Sum  Commented=on
  Constant : Constant  Value=R_wheel
  Constant1 : Constant  Value=inf
  Constant2 : Constant
  Constant3 : Constant  Value=0
  Constant4 : Constant  Commented=on
  Divide : Product  Inputs=*/
  From : From  Commented=on  GotoTag=SL
  From1 : From  Commented=on  GotoTag=SS
  Product : Product
  Product3 : Product  Commented=on
  Product4 : Product  Commented=on
  Sqrt : Sqrt  Commented=on
  Subtract : Sum  Inputs=+-
  Switch : Switch  Criteria=u2 ~= 0  SaturateOnIntegerOverflow=off  InputSameDT=off
  Switch1 : Switch  Criteria=u2 > Threshold  Threshold=1  SaturateOnIntegerOverflow=off  InputSameDT=off
  Switch2 : Switch  Commented=on  Criteria=u2 > Threshold  Threshold=1  SaturateOnIntegerOverflow=off  InputSameDT=off
  Switch3 : Switch  Criteria=u2 > Threshold  SaturateOnIntegerOverflow=off  InputSameDT=off
  SL : Outport
  wires:
  Switch/1 -> Divide/2
  Constant1/1 -> Switch/3
  Subtract/1 -> Divide/1
  Corner Speed/1 -> Subtract/2
  Add/1 -> Sqrt/1
  Sqrt/1 -> Switch2/2, Switch2/1
  Constant4/1 -> Switch2/3
  From/1 -> Product3/1, Product3/2
  Product4/1 -> Add/2
  From1/1 -> Product4/2, Product4/1
  Product3/1 -> Add/1
  Constant/1 -> Product/2
  Wheel Omega1/1 -> Product/1
  Product/1 -> Subtract/1, Switch/1, Switch/2  "Omega * Rw"
  Constant2/1 -> Switch1/1
  Divide/1 -> Switch3/2, Switch3/1  "Longitudinal Slip (SL)"
  Constant3/1 -> Switch3/3
  Switch3/1 -> Switch1/3, Switch1/2
  Switch1/1 -> SL/1

== system FullCarLateral/Car/Longitudinal Slip/Longitudinal Slip Calc FL2/Brake Calc ==
  Wheel Omega : Inport
  Corner Speed : Inport  Port=2
  Action Port : ActionPort  ActionPortLabel=elseif(u1 < 0)
  Abs : Abs  SaturateOnIntegerOverflow=off
  Abs1 : Abs  SaturateOnIntegerOverflow=off
  Add : Sum  Commented=on
  Constant : Constant  Value=R_wheel
  Constant1 : Constant  Value=-1
  Constant2 : Constant  Commented=on  Value=-1
  Constant3 : Constant  Commented=on
  Divide : Product  Inputs=*/
  From : From  Commented=on  GotoTag=SL
  From1 : From  Commented=on  GotoTag=SS
  Gain : Gain  Gain=-1
  Goto : Goto  Commented=on  GotoTag=SL
  Goto1 : Goto  Commented=on  GotoTag=SS
  Product : Product
  Product3 : Product  Commented=on
  Product4 : Product  Commented=on
  Product5 : Product  Commented=on
  Sqrt : Sqrt  Commented=on
  Subtract : Sum  Inputs=+-
  Switch : Switch  Criteria=u2 > Threshold  Threshold=1  SaturateOnIntegerOverflow=off  InputSameDT=off
  Switch1 : Switch  Commented=on  Criteria=u2 > Threshold  Threshold=1  SaturateOnIntegerOverflow=off  InputSameDT=off
  SL : Outport
  wires:
  Divide/1 -> Switch/3, Abs/1  "Longitudinal Slip (SL)"
  Subtract/1 -> Divide/1
  Product/1 -> Subtract/1  "Omega * Rw"
  Corner Speed/1 -> Subtract/2, Divide/2
  Wheel Omega/1 -> Product/1
  Constant/1 -> Product/2
  Abs/1 -> Switch/2
  Switch/1 -> Abs1/1, Goto/1
  From/1 -> Product3/1, Product3/2
  From1/1 -> Product4/2, Product4/1
  Product3/1 -> Add/1
  Product4/1 -> Add/2
  Add/1 -> Sqrt/1
  Constant2/1 -> Product5/2
  Sqrt/1 -> Switch1/2, Switch1/1
  Constant3/1 -> Switch1/3
  Switch1/1 -> Product5/1
  Constant1/1 -> Switch/1
  Gain/1 -> SL/1
  Abs1/1 -> Gain/1

== system FullCarLateral/Car/Longitudinal Slip/Longitudinal Slip Calc FL2/If Action Subsystem ==
  Corner Speed : Inport
  Action Port : ActionPort  ActionPortLabel=else
  Out1 : Outport
  wires:
  Corner Speed/1 -> Out1/1

== system FullCarLateral/Car/Longitudinal Slip/Longitudinal Slip Calc FL3/Accel. Calc ==
  Corner Speed : Inport
  Wheel Omega1 : Inport  Port=2
  Action Port : ActionPort  ActionPortLabel=if(u1 > 0)
  Add : Sum  Commented=on
  Constant : Constant  Value=R_wheel
  Constant1 : Constant  Value=inf
  Constant2 : Constant
  Constant3 : Constant  Value=0
  Constant4 : Constant  Commented=on
  Divide : Product  Inputs=*/
  From : From  Commented=on  GotoTag=SL
  From1 : From  Commented=on  GotoTag=SS
  Product : Product
  Product3 : Product  Commented=on
  Product4 : Product  Commented=on
  Sqrt : Sqrt  Commented=on
  Subtract : Sum  Inputs=+-
  Switch : Switch  Criteria=u2 ~= 0  SaturateOnIntegerOverflow=off  InputSameDT=off
  Switch1 : Switch  Criteria=u2 > Threshold  Threshold=1  SaturateOnIntegerOverflow=off  InputSameDT=off
  Switch2 : Switch  Commented=on  Criteria=u2 > Threshold  Threshold=1  SaturateOnIntegerOverflow=off  InputSameDT=off
  Switch3 : Switch  Criteria=u2 > Threshold  SaturateOnIntegerOverflow=off  InputSameDT=off
  SL : Outport
  wires:
  Switch1/1 -> SL/1
  Switch3/1 -> Switch1/2, Switch1/3
  Constant3/1 -> Switch3/3
  Divide/1 -> Switch3/1, Switch3/2  "Longitudinal Slip (SL)"
  Constant2/1 -> Switch1/1
  Product/1 -> Switch/2, Switch/1, Subtract/1  "Omega * Rw"
  Wheel Omega1/1 -> Product/1
  Constant/1 -> Product/2
  Product3/1 -> Add/1
  From1/1 -> Product4/1, Product4/2
  Product4/1 -> Add/2
  From/1 -> Product3/2, Product3/1
  Constant4/1 -> Switch2/3
  Sqrt/1 -> Switch2/1, Switch2/2
  Add/1 -> Sqrt/1
  Corner Speed/1 -> Subtract/2
  Subtract/1 -> Divide/1
  Constant1/1 -> Switch/3
  Switch/1 -> Divide/2

== system FullCarLateral/Car/Longitudinal Slip/Longitudinal Slip Calc FL3/Brake Calc ==
  Wheel Omega : Inport
  Corner Speed : Inport  Port=2
  Action Port : ActionPort  ActionPortLabel=elseif(u1 < 0)
  Abs : Abs  SaturateOnIntegerOverflow=off
  Abs1 : Abs  SaturateOnIntegerOverflow=off
  Add : Sum  Commented=on
  Constant : Constant  Value=R_wheel
  Constant1 : Constant  Value=-1
  Constant2 : Constant  Commented=on  Value=-1
  Constant3 : Constant  Commented=on
  Divide : Product  Inputs=*/
  From : From  Commented=on  GotoTag=SL
  From1 : From  Commented=on  GotoTag=SS
  Gain : Gain  Gain=-1
  Goto : Goto  Commented=on  GotoTag=SL
  Goto1 : Goto  Commented=on  GotoTag=SS
  Product : Product
  Product3 : Product  Commented=on
  Product4 : Product  Commented=on
  Product5 : Product  Commented=on
  Sqrt : Sqrt  Commented=on
  Subtract : Sum  Inputs=+-
  Switch : Switch  Criteria=u2 > Threshold  Threshold=1  SaturateOnIntegerOverflow=off  InputSameDT=off
  Switch1 : Switch  Commented=on  Criteria=u2 > Threshold  Threshold=1  SaturateOnIntegerOverflow=off  InputSameDT=off
  SL : Outport
  wires:
  Abs1/1 -> Gain/1
  Gain/1 -> SL/1
  Constant1/1 -> Switch/1
  Switch1/1 -> Product5/1
  Constant3/1 -> Switch1/3
  Sqrt/1 -> Switch1/1, Switch1/2
  Constant2/1 -> Product5/2
  Add/1 -> Sqrt/1
  Product4/1 -> Add/2
  Product3/1 -> Add/1
  From1/1 -> Product4/1, Product4/2
  From/1 -> Product3/2, Product3/1
  Switch/1 -> Goto/1, Abs1/1
  Abs/1 -> Switch/2
  Constant/1 -> Product/2
  Wheel Omega/1 -> Product/1
  Corner Speed/1 -> Divide/2, Subtract/2
  Product/1 -> Subtract/1  "Omega * Rw"
  Subtract/1 -> Divide/1
  Divide/1 -> Abs/1, Switch/3  "Longitudinal Slip (SL)"

== system FullCarLateral/Car/Longitudinal Slip/Longitudinal Slip Calc FL3/If Action Subsystem ==
  Corner Speed : Inport
  Action Port : ActionPort  ActionPortLabel=else
  Out1 : Outport
  wires:
  Corner Speed/1 -> Out1/1

== system FullCarLateral/Car/Tire Model Pacejka 5.2/FY DIRECTIONAL CONSTRAIN FL/If Action Subsystem ==
  In1 : Inport
  Action Port : ActionPort  ActionPortLabel=else
  Out1 : Outport
  wires:
  In1/1 -> Out1/1

== system FullCarLateral/Car/Tire Model Pacejka 5.2/FY DIRECTIONAL CONSTRAIN FL/NEGATIVE FY ==
  In1 : Inport
  Action Port : ActionPort  ActionPortLabel=elseif(u1 > 0)
  Abs : Abs  SaturateOnIntegerOverflow=off
  Gain : Gain  Gain=-1
  Out1 : Outport
  wires:
  In1/1 -> Abs/1
  Abs/1 -> Gain/1
  Gain/1 -> Out1/1

== system FullCarLateral/Car/Tire Model Pacejka 5.2/FY DIRECTIONAL CONSTRAIN FL/POSITIVE FY ==
  In1 : Inport
  Action Port : ActionPort  ActionPortLabel=if(u1 < 0)
  Abs : Abs  SaturateOnIntegerOverflow=off
  Out1 : Outport
  wires:
  In1/1 -> Abs/1
  Abs/1 -> Out1/1

== system FullCarLateral/Car/Tire Model Pacejka 5.2/FY DIRECTIONAL CONSTRAIN FR/If Action Subsystem ==
  In1 : Inport
  Action Port : ActionPort  ActionPortLabel=else
  Out1 : Outport
  wires:
  In1/1 -> Out1/1

== system FullCarLateral/Car/Tire Model Pacejka 5.2/FY DIRECTIONAL CONSTRAIN FR/NEGATIVE FY ==
  In1 : Inport
  Action Port : ActionPort  ActionPortLabel=elseif(u1 > 0)
  Abs : Abs  SaturateOnIntegerOverflow=off
  Gain : Gain  Gain=-1
  Out1 : Outport
  wires:
  Gain/1 -> Out1/1
  Abs/1 -> Gain/1
  In1/1 -> Abs/1

== system FullCarLateral/Car/Tire Model Pacejka 5.2/FY DIRECTIONAL CONSTRAIN FR/POSITIVE FY ==
  In1 : Inport
  Action Port : ActionPort  ActionPortLabel=if(u1 < 0)
  Abs : Abs  SaturateOnIntegerOverflow=off
  Out1 : Outport
  wires:
  Abs/1 -> Out1/1
  In1/1 -> Abs/1

== system FullCarLateral/Car/Tire Model Pacejka 5.2/FY DIRECTIONAL CONSTRAIN RL/If Action Subsystem ==
  In1 : Inport
  Action Port : ActionPort  ActionPortLabel=else
  Out1 : Outport
  wires:
  In1/1 -> Out1/1

== system FullCarLateral/Car/Tire Model Pacejka 5.2/FY DIRECTIONAL CONSTRAIN RL/NEGATIVE FY ==
  In1 : Inport
  Action Port : ActionPort  ActionPortLabel=elseif(u1 > 0)
  Abs : Abs  SaturateOnIntegerOverflow=off
  Gain : Gain  Gain=-1
  Out1 : Outport
  wires:
  In1/1 -> Abs/1
  Abs/1 -> Gain/1
  Gain/1 -> Out1/1

== system FullCarLateral/Car/Tire Model Pacejka 5.2/FY DIRECTIONAL CONSTRAIN RL/POSITIVE FY ==
  In1 : Inport
  Action Port : ActionPort  ActionPortLabel=if(u1 < 0)
  Abs : Abs  SaturateOnIntegerOverflow=off
  Out1 : Outport
  wires:
  In1/1 -> Abs/1
  Abs/1 -> Out1/1

== system FullCarLateral/Car/Tire Model Pacejka 5.2/FY DIRECTIONAL CONSTRAIN RR/If Action Subsystem ==
  In1 : Inport
  Action Port : ActionPort  ActionPortLabel=else
  Out1 : Outport
  wires:
  In1/1 -> Out1/1

== system FullCarLateral/Car/Tire Model Pacejka 5.2/FY DIRECTIONAL CONSTRAIN RR/NEGATIVE FY ==
  In1 : Inport
  Action Port : ActionPort  ActionPortLabel=elseif(u1 > 0)
  Abs : Abs  SaturateOnIntegerOverflow=off
  Gain : Gain  Gain=-1
  Out1 : Outport
  wires:
  Gain/1 -> Out1/1
  Abs/1 -> Gain/1
  In1/1 -> Abs/1

== system FullCarLateral/Car/Tire Model Pacejka 5.2/FY DIRECTIONAL CONSTRAIN RR/POSITIVE FY ==
  In1 : Inport
  Action Port : ActionPort  ActionPortLabel=if(u1 < 0)
  Abs : Abs  SaturateOnIntegerOverflow=off
  Out1 : Outport
  wires:
  Abs/1 -> Out1/1
  In1/1 -> Abs/1

== system FullCarLateral/Car/Tire Model Pacejka 5.2/Subsystem/If Action Subsystem ==
  FX : Inport
  Action Port : ActionPort  ActionPortLabel=if(u1 >= 0)
  Gain8 : Gain  Gain=tireFactor_X_Accel
  Out1 : Outport
  wires:
  FX/1 -> Gain8/1
  Gain8/1 -> Out1/1

== system FullCarLateral/Car/Tire Model Pacejka 5.2/Subsystem/If Action Subsystem1 ==
  FX : Inport
  Action Port : ActionPort  ActionPortLabel=else
  Gain : Gain  Gain=tireFactor_X_Brake
  Out1 : Outport
  wires:
  FX/1 -> Gain/1
  Gain/1 -> Out1/1

== system FullCarLateral/Car/Tire Model Pacejka 5.2/Subsystem1/If Action Subsystem ==
  FX : Inport
  Action Port : ActionPort  ActionPortLabel=if(u1 >= 0)
  Gain8 : Gain  Gain=tireFactor_X_Accel
  Out1 : Outport
  wires:
  Gain8/1 -> Out1/1
  FX/1 -> Gain8/1

== system FullCarLateral/Car/Tire Model Pacejka 5.2/Subsystem1/If Action Subsystem1 ==
  FX : Inport
  Action Port : ActionPort  ActionPortLabel=else
  Gain : Gain  Gain=tireFactor_X_Brake
  Out1 : Outport
  wires:
  Gain/1 -> Out1/1
  FX/1 -> Gain/1

== system FullCarLateral/Car/Tire Model Pacejka 5.2/Subsystem2/If Action Subsystem ==
  FX : Inport
  Action Port : ActionPort  ActionPortLabel=if(u1 >= 0)
  Gain8 : Gain  Gain=tireFactor_X_Accel
  Out1 : Outport
  wires:
  FX/1 -> Gain8/1
  Gain8/1 -> Out1/1

== system FullCarLateral/Car/Tire Model Pacejka 5.2/Subsystem2/If Action Subsystem1 ==
  FX : Inport
  Action Port : ActionPort  ActionPortLabel=else
  Gain : Gain  Gain=tireFactor_X_Brake
  Out1 : Outport
  wires:
  FX/1 -> Gain/1
  Gain/1 -> Out1/1

== system FullCarLateral/Car/Tire Model Pacejka 5.2/Subsystem3/If Action Subsystem ==
  FX : Inport
  Action Port : ActionPort  ActionPortLabel=if(u1 >= 0)
  Gain8 : Gain  Gain=tireFactor_X_Accel
  Out1 : Outport
  wires:
  Gain8/1 -> Out1/1
  FX/1 -> Gain8/1

== system FullCarLateral/Car/Tire Model Pacejka 5.2/Subsystem3/If Action Subsystem1 ==
  FX : Inport
  Action Port : ActionPort  ActionPortLabel=else
  Gain : Gain  Gain=tireFactor_X_Brake
  Out1 : Outport
  wires:
  Gain/1 -> Out1/1
  FX/1 -> Gain/1

== system FullCarLateral/Car/Wheel Dynamics/Subsystem4/Accel. or Rolling No Slip ==
  Requested Motor Torque : Inport
  FX Resistance : Inport  Port=2
  Long Corner Vel : Inport  Port=3
  Action Port : ActionPort  ActionPortLabel=if(u1 >= 0)
  Accelerating : Subsystem  TreatAsAtomicUnit=on
  If : If  IfExpression=u1 > rollingNoSlipTorqueThreshold
  Merge : Merge
  Merge1 : Merge
  Rolling No Slip : Subsystem  TreatAsAtomicUnit=on
  Wheel Omega : Outport
  Constrained Motor Torque : Outport  Port=2
  wires:
  Requested Motor Torque/1 -> Rolling No Slip/2(Requested Motor Torque), Accelerating/1(Requested Motor Torque), If/1
  If/1 -> Accelerating/Action
  If/2 -> Rolling No Slip/Action
  Accelerating/1(Accelerating Wheel Omega) -> Merge/1
  Rolling No Slip/1(No Slip Wheel Omega) -> Merge/2
  Merge/1 -> Wheel Omega/1
  Long Corner Vel/1 -> Rolling No Slip/1(Long Corner Vel)
  FX Resistance/1 -> Accelerating/2(FX Resistance)
  Accelerating/2(Constrained Motor Torque) -> Merge1/1
  Rolling No Slip/2(Constrained Motor Torque) -> Merge1/2
  Merge1/1 -> Constrained Motor Torque/1

== system FullCarLateral/Car/Wheel Dynamics/Subsystem4/Braking ==
  Requested Motor Torque : Inport
  FX Resistance : Inport  Port=2
  Action Port : ActionPort  ActionPortLabel=else
  Constant : Constant  Value=0
  Motor Omega Calc : Subsystem
  Switch : Switch  Criteria=u2 > Threshold  SaturateOnIntegerOverflow=off  InputSameDT=off
  Wheel Omega : Outport
  Constrained Motor Torque : Outport  Port=2
  wires:
  Requested Motor Torque/1 -> Constrained Motor Torque/1, Motor Omega Calc/1(Motor Torque)
  FX Resistance/1 -> Motor Omega Calc/2(FX Resistance)
  Motor Omega Calc/1(Wheel Omega) -> Switch/2, Switch/1
  Switch/1 -> Wheel Omega/1
  Constant/1 -> Switch/3

== system FullCarLateral/Car/Wheel Dynamics/Subsystem5/Accel. or Rolling No Slip ==
  Requested Motor Torque : Inport
  FX Resistance : Inport  Port=2
  Long Corner Vel : Inport  Port=3
  Action Port : ActionPort  ActionPortLabel=if(u1 >= 0)
  Accelerating : Subsystem  TreatAsAtomicUnit=on
  If : If  IfExpression=u1 > rollingNoSlipTorqueThreshold
  Merge : Merge
  Merge1 : Merge
  Rolling No Slip : Subsystem  TreatAsAtomicUnit=on
  Wheel Omega : Outport
  Constrained Motor Torque : Outport  Port=2
  wires:
  Merge1/1 -> Constrained Motor Torque/1
  Rolling No Slip/2(Constrained Motor Torque) -> Merge1/2
  Accelerating/2(Constrained Motor Torque) -> Merge1/1
  FX Resistance/1 -> Accelerating/2(FX Resistance)
  Long Corner Vel/1 -> Rolling No Slip/1(Long Corner Vel)
  Merge/1 -> Wheel Omega/1
  Rolling No Slip/1(No Slip Wheel Omega) -> Merge/2
  Accelerating/1(Accelerating Wheel Omega) -> Merge/1
  If/2 -> Rolling No Slip/Action
  If/1 -> Accelerating/Action
  Requested Motor Torque/1 -> If/1, Rolling No Slip/2(Requested Motor Torque), Accelerating/1(Requested Motor Torque)

== system FullCarLateral/Car/Wheel Dynamics/Subsystem5/Braking ==
  Requested Motor Torque : Inport
  FX Resistance : Inport  Port=2
  Action Port : ActionPort  ActionPortLabel=else
  Constant : Constant  Value=0
  Motor Omega Calc : Subsystem
  Switch : Switch  Criteria=u2 > Threshold  SaturateOnIntegerOverflow=off  InputSameDT=off
  Wheel Omega : Outport
  Constrained Motor Torque : Outport  Port=2
  wires:
  Constant/1 -> Switch/3
  Switch/1 -> Wheel Omega/1
  Motor Omega Calc/1(Wheel Omega) -> Switch/1, Switch/2
  FX Resistance/1 -> Motor Omega Calc/2(FX Resistance)
  Requested Motor Torque/1 -> Motor Omega Calc/1(Motor Torque), Constrained Motor Torque/1

== system FullCarLateral/Car/Wheel Dynamics/Subsystem6/Accel. or Rolling No Slip ==
  Requested Motor Torque : Inport
  FX Resistance : Inport  Port=2
  Long Corner Vel : Inport  Port=3
  Action Port : ActionPort  ActionPortLabel=if(u1 >= 0)
  Accelerating : Subsystem  TreatAsAtomicUnit=on
  If : If  IfExpression=u1 > rollingNoSlipTorqueThreshold
  Merge : Merge
  Merge1 : Merge
  Rolling No Slip : Subsystem  TreatAsAtomicUnit=on
  Wheel Omega : Outport
  Constrained Motor Torque : Outport  Port=2
  wires:
  Requested Motor Torque/1 -> Rolling No Slip/2(Requested Motor Torque), Accelerating/1(Requested Motor Torque), If/1
  If/1 -> Accelerating/Action
  If/2 -> Rolling No Slip/Action
  Accelerating/1(Accelerating Wheel Omega) -> Merge/1
  Rolling No Slip/1(No Slip Wheel Omega) -> Merge/2
  Merge/1 -> Wheel Omega/1
  Long Corner Vel/1 -> Rolling No Slip/1(Long Corner Vel)
  FX Resistance/1 -> Accelerating/2(FX Resistance)
  Accelerating/2(Constrained Motor Torque) -> Merge1/1
  Rolling No Slip/2(Constrained Motor Torque) -> Merge1/2
  Merge1/1 -> Constrained Motor Torque/1

== system FullCarLateral/Car/Wheel Dynamics/Subsystem6/Braking ==
  Requested Motor Torque : Inport
  FX Resistance : Inport  Port=2
  Action Port : ActionPort  ActionPortLabel=else
  Constant : Constant  Value=0
  Motor Omega Calc : Subsystem
  Switch : Switch  Criteria=u2 > Threshold  SaturateOnIntegerOverflow=off  InputSameDT=off
  Wheel Omega : Outport
  Constrained Motor Torque : Outport  Port=2
  wires:
  Requested Motor Torque/1 -> Constrained Motor Torque/1, Motor Omega Calc/1(Motor Torque)
  FX Resistance/1 -> Motor Omega Calc/2(FX Resistance)
  Motor Omega Calc/1(Wheel Omega) -> Switch/2, Switch/1
  Switch/1 -> Wheel Omega/1
  Constant/1 -> Switch/3
